simulink library "halin"  (R2021b)
settings: Solver=VariableStepAuto  StartTime=0.0  StopTime=10.0  RelTol=1e-3
undefined symbols (not defined in the file): TRUE
libraries: FVT_lib x177, hcu_lib x55
(part 11 of 17)

== system halin/HAL_IN/CAN4/ZONE_L1 ==
  DT_CAN4_SG_ZONE_L1 : Inport
  ZLDSEATAntiSta : Subsystem
  ZLDSEATEntryFunSta : Subsystem
  ZLDSEATErrorSta : Subsystem
  ZLDSEATMemSetSta : Subsystem
  ZLDSEATModeSta : Subsystem
  ZLDSEATVentSta : Subsystem
  ZLDSEATheaterSta : Subsystem
  bus_selector : BusSelector  OutputSignals=CAN4_ZL_DSEAT_Anti_Sta
  bus_selector1 : BusSelector  OutputSignals=CAN4_ZL_DSEAT_EntryFun_Sta
  bus_selector2 : BusSelector  OutputSignals=CAN4_ZL_DSEAT_Error_Sta
  bus_selector3 : BusSelector  OutputSignals=CAN4_ZL_DSEAT_MemSet_Sta
  bus_selector4 : BusSelector  OutputSignals=CAN4_ZL_DSEAT_Mode_Sta
  bus_selector5 : BusSelector  OutputSignals=CAN4_ZL_DSEAT_Vent_Sta
  bus_selector6 : BusSelector  OutputSignals=CAN4_ZL_DSEAT_heater_Sta
  VHAL_ZLDSEATAntiSta_flg : Outport
  VHAL_ZLDSEATEntryFunSta_flg : Outport  Port=2
  VHAL_ZLDSEATErrorSta_flg : Outport  Port=3
  VHAL_ZLDSEATMemSetSta_enum : Outport  Port=4
  VHAL_ZLDSEATModeSta_enum : Outport  Port=5
  VHAL_ZLDSEATVentSta_enum : Outport  Port=6
  VHAL_ZLDSEATheaterSta_enum : Outport  Port=7
  wires:
  DT_CAN4_SG_ZONE_L1/1 -> [DT_CAN4_SG_ZONE_L1]
  [DT_CAN4_SG_ZONE_L1] -> bus_selector/1
  bus_selector/1 -> ZLDSEATAntiSta/1(ZL_DSEAT_Anti_Sta)  "<CAN4_ZL_DSEAT_Anti_Sta>"
  ZLDSEATAntiSta/1(VHAL_ZLDSEATAntiSta_flg) -> VHAL_ZLDSEATAntiSta_flg/1
  [DT_CAN4_SG_ZONE_L1] -> bus_selector1/1
  bus_selector1/1 -> ZLDSEATEntryFunSta/1(ZL_DSEAT_EntryFun_Sta)  "<CAN4_ZL_DSEAT_EntryFun_Sta>"
  ZLDSEATEntryFunSta/1(VHAL_ZLDSEATEntryFunSta_flg) -> VHAL_ZLDSEATEntryFunSta_flg/1
  [DT_CAN4_SG_ZONE_L1] -> bus_selector2/1
  bus_selector2/1 -> ZLDSEATErrorSta/1(ZL_DSEAT_Error_Sta)  "<CAN4_ZL_DSEAT_Error_Sta>"
  ZLDSEATErrorSta/1(VHAL_ZLDSEATErrorSta_flg) -> VHAL_ZLDSEATErrorSta_flg/1
  [DT_CAN4_SG_ZONE_L1] -> bus_selector3/1
  bus_selector3/1 -> ZLDSEATMemSetSta/1(ZL_DSEAT_MemSet_Sta)  "<CAN4_ZL_DSEAT_MemSet_Sta>"
  ZLDSEATMemSetSta/1(VHAL_ZLDSEATMemSetSta_enum) -> VHAL_ZLDSEATMemSetSta_enum/1
  [DT_CAN4_SG_ZONE_L1] -> bus_selector4/1
  bus_selector4/1 -> ZLDSEATModeSta/1(ZL_DSEAT_Mode_Sta)  "<CAN4_ZL_DSEAT_Mode_Sta>"
  ZLDSEATModeSta/1(VHAL_ZLDSEATModeSta_enum) -> VHAL_ZLDSEATModeSta_enum/1
  [DT_CAN4_SG_ZONE_L1] -> bus_selector5/1
  bus_selector5/1 -> ZLDSEATVentSta/1(ZL_DSEAT_Vent_Sta)  "<CAN4_ZL_DSEAT_Vent_Sta>"
  ZLDSEATVentSta/1(VHAL_ZLDSEATVentSta_enum) -> VHAL_ZLDSEATVentSta_enum/1
  [DT_CAN4_SG_ZONE_L1] -> bus_selector6/1
  bus_selector6/1 -> ZLDSEATheaterSta/1(ZL_DSEAT_heater_Sta)  "<CAN4_ZL_DSEAT_heater_Sta>"
  ZLDSEATheaterSta/1(VHAL_ZLDSEATheaterSta_enum) -> VHAL_ZLDSEATheaterSta_enum/1

== system halin/HAL_IN/CAN4/ZONE_L2 ==
  DT_CAN4_SG_ZONE_L2 : Inport
  ZLAPMWinLFOpenedSta : Subsystem
  ZLAPMWinLROpenedSta : Subsystem
  bus_selector : BusSelector  OutputSignals=CAN4_ZL_APM_WinLFOpened_Sta
  bus_selector1 : BusSelector  OutputSignals=CAN4_ZL_APM_WinLROpened_Sta
  VHAL_ZLAPMWinLFOpenedSta_pct : Outport
  VHAL_ZLAPMWinLROpenedSta_pct : Outport  Port=2
  wires:
  DT_CAN4_SG_ZONE_L2/1 -> [DT_CAN4_SG_ZONE_L2]
  [DT_CAN4_SG_ZONE_L2] -> bus_selector/1
  bus_selector/1 -> ZLAPMWinLFOpenedSta/1(ZL_APM_WinLFOpened_Sta)  "<CAN4_ZL_APM_WinLFOpened_Sta>"
  ZLAPMWinLFOpenedSta/1(VHAL_ZLAPMWinLFOpenedSta_pct) -> VHAL_ZLAPMWinLFOpenedSta_pct/1
  [DT_CAN4_SG_ZONE_L2] -> bus_selector1/1
  bus_selector1/1 -> ZLAPMWinLROpenedSta/1(ZL_APM_WinLROpened_Sta)  "<CAN4_ZL_APM_WinLROpened_Sta>"
  ZLAPMWinLROpenedSta/1(VHAL_ZLAPMWinLROpenedSta_pct) -> VHAL_ZLAPMWinLROpenedSta_pct/1

== system halin/HAL_IN/CAN4/ZONE_R1 ==
  DT_CAN4_SG_ZONE_R1 : Inport
  ZRPSEATErrorSta : Subsystem
  ZRPSEATModeSta : Subsystem
  ZRPSEATVentSta : Subsystem
  ZRPSEATheaterSta : Subsystem
  ZRPTGActiveSta : Subsystem
  ZRPTGExistSta : Subsystem
  ZRPTGIsSetHeightSta : Subsystem
  ZRPTGSysSta : Subsystem
  bus_selector : BusSelector  OutputSignals=CAN4_ZR_PSEAT_Error_Sta
  bus_selector1 : BusSelector  OutputSignals=CAN4_ZR_PSEAT_Mode_Sta
  bus_selector2 : BusSelector  OutputSignals=CAN4_ZR_PSEAT_Vent_Sta
  bus_selector3 : BusSelector  OutputSignals=CAN4_ZR_PSEAT_heater_Sta
  bus_selector4 : BusSelector  OutputSignals=CAN4_ZR_PTG_Active_Sta
  bus_selector5 : BusSelector  OutputSignals=CAN4_ZR_PTG_Exist_Sta
  bus_selector6 : BusSelector  OutputSignals=CAN4_ZR_PTG_IsSetHeight_Sta
  bus_selector7 : BusSelector  OutputSignals=CAN4_ZR_PTG_Sys_Sta
  VHAL_ZRPSEATErrorSta_flg : Outport
  VHAL_ZRPSEATModeSta_enum : Outport  Port=2
  VHAL_ZRPSEATVentSta_enum : Outport  Port=3
  VHAL_ZRPSEATheaterSta_enum : Outport  Port=4
  VHAL_ZRPTGActiveSta_enum : Outport  Port=5
  VHAL_ZRPTGExistSta_flg : Outport  Port=6
  VHAL_ZRPTGIsSetHeightSta_flg : Outport  Port=7
  VHAL_ZRPTGSysSta_enum : Outport  Port=8
  wires:
  DT_CAN4_SG_ZONE_R1/1 -> [DT_CAN4_SG_ZONE_R1]
  [DT_CAN4_SG_ZONE_R1] -> bus_selector/1
  bus_selector/1 -> ZRPSEATErrorSta/1(ZR_PSEAT_Error_Sta)  "<CAN4_ZR_PSEAT_Error_Sta>"
  ZRPSEATErrorSta/1(VHAL_ZRPSEATErrorSta_flg) -> VHAL_ZRPSEATErrorSta_flg/1
  [DT_CAN4_SG_ZONE_R1] -> bus_selector1/1
  bus_selector1/1 -> ZRPSEATModeSta/1(ZR_PSEAT_Mode_Sta)  "<CAN4_ZR_PSEAT_Mode_Sta>"
  ZRPSEATModeSta/1(VHAL_ZRPSEATModeSta_enum) -> VHAL_ZRPSEATModeSta_enum/1
  [DT_CAN4_SG_ZONE_R1] -> bus_selector2/1
  bus_selector2/1 -> ZRPSEATVentSta/1(ZR_PSEAT_Vent_Sta)  "<CAN4_ZR_PSEAT_Vent_Sta>"
  ZRPSEATVentSta/1(VHAL_ZRPSEATVentSta_enum) -> VHAL_ZRPSEATVentSta_enum/1
  [DT_CAN4_SG_ZONE_R1] -> bus_selector3/1
  bus_selector3/1 -> ZRPSEATheaterSta/1(ZR_PSEAT_heater_Sta)  "<CAN4_ZR_PSEAT_heater_Sta>"
  ZRPSEATheaterSta/1(VHAL_ZRPSEATheaterSta_enum) -> VHAL_ZRPSEATheaterSta_enum/1
  [DT_CAN4_SG_ZONE_R1] -> bus_selector4/1
  bus_selector4/1 -> ZRPTGActiveSta/1(ZR_PTG_Active_Sta)  "<CAN4_ZR_PTG_Active_Sta>"
  ZRPTGActiveSta/1(VHAL_ZRPTGActiveSta_enum) -> VHAL_ZRPTGActiveSta_enum/1
  [DT_CAN4_SG_ZONE_R1] -> bus_selector5/1
  bus_selector5/1 -> ZRPTGExistSta/1(ZR_PTG_Exist_Sta)  "<CAN4_ZR_PTG_Exist_Sta>"
  ZRPTGExistSta/1(VHAL_ZRPTGExistSta_flg) -> VHAL_ZRPTGExistSta_flg/1
  [DT_CAN4_SG_ZONE_R1] -> bus_selector6/1
  bus_selector6/1 -> ZRPTGIsSetHeightSta/1(ZR_PTG_IsSetHeight_Sta)  "<CAN4_ZR_PTG_IsSetHeight_Sta>"
  ZRPTGIsSetHeightSta/1(VHAL_ZRPTGIsSetHeightSta_flg) -> VHAL_ZRPTGIsSetHeightSta_flg/1
  [DT_CAN4_SG_ZONE_R1] -> bus_selector7/1
  bus_selector7/1 -> ZRPTGSysSta/1(ZR_PTG_Sys_Sta)  "<CAN4_ZR_PTG_Sys_Sta>"
  ZRPTGSysSta/1(VHAL_ZRPTGSysSta_enum) -> VHAL_ZRPTGSysSta_enum/1

== system halin/HAL_IN/CAN4/ZONE_R2 ==
  DT_CAN4_SG_ZONE_R2 : Inport
  ZRAPMWinRFOpenedSta : Subsystem
  ZRAPMWinRROpenedSta : Subsystem
  ZRSEATLVentSta : Subsystem
  ZRSEATMLVentSta : Subsystem
  ZRSEATMRVentSta : Subsystem
  ZRSEATRVentSta : Subsystem
  bus_selector : BusSelector  OutputSignals=CAN4_ZR_APM_WinRFOpened_Sta
  bus_selector1 : BusSelector  OutputSignals=CAN4_ZR_APM_WinRROpened_Sta
  bus_selector2 : BusSelector  OutputSignals=CAN4_ZR_SEAT_LVent_Sta
  bus_selector3 : BusSelector  OutputSignals=CAN4_ZR_SEAT_MLVent_Sta
  bus_selector4 : BusSelector  OutputSignals=CAN4_ZR_SEAT_MRVent_Sta
  bus_selector5 : BusSelector  OutputSignals=CAN4_ZR_SEAT_RVent_Sta
  VHAL_ZRAPMWinRFOpenedSta_pct : Outport
  VHAL_ZRAPMWinRROpenedSta_pct : Outport  Port=2
  VHAL_ZRSEATLVentSta_enum : Outport  Port=3
  VHAL_ZRSEATMLVentSta_enum : Outport  Port=4
  VHAL_ZRSEATMRVentSta_enum : Outport  Port=5
  VHAL_ZRSEATRVentSta_enum : Outport  Port=6
  wires:
  DT_CAN4_SG_ZONE_R2/1 -> [DT_CAN4_SG_ZONE_R2]
  [DT_CAN4_SG_ZONE_R2] -> bus_selector/1
  bus_selector/1 -> ZRAPMWinRFOpenedSta/1(ZR_APM_WinRFOpened_Sta)  "<CAN4_ZR_APM_WinRFOpened_Sta>"
  ZRAPMWinRFOpenedSta/1(VHAL_ZRAPMWinRFOpenedSta_pct) -> VHAL_ZRAPMWinRFOpenedSta_pct/1
  [DT_CAN4_SG_ZONE_R2] -> bus_selector1/1
  bus_selector1/1 -> ZRAPMWinRROpenedSta/1(ZR_APM_WinRROpened_Sta)  "<CAN4_ZR_APM_WinRROpened_Sta>"
  ZRAPMWinRROpenedSta/1(VHAL_ZRAPMWinRROpenedSta_pct) -> VHAL_ZRAPMWinRROpenedSta_pct/1
  [DT_CAN4_SG_ZONE_R2] -> bus_selector2/1
  bus_selector2/1 -> ZRSEATLVentSta/1(ZR_SEAT_LVent_Sta)  "<CAN4_ZR_SEAT_LVent_Sta>"
  ZRSEATLVentSta/1(VHAL_ZRSEATLVentSta_enum) -> VHAL_ZRSEATLVentSta_enum/1
  [DT_CAN4_SG_ZONE_R2] -> bus_selector3/1
  bus_selector3/1 -> ZRSEATMLVentSta/1(ZR_SEAT_MLVent_Sta)  "<CAN4_ZR_SEAT_MLVent_Sta>"
  ZRSEATMLVentSta/1(VHAL_ZRSEATMLVentSta_enum) -> VHAL_ZRSEATMLVentSta_enum/1
  [DT_CAN4_SG_ZONE_R2] -> bus_selector4/1
  bus_selector4/1 -> ZRSEATMRVentSta/1(ZR_SEAT_MRVent_Sta)  "<CAN4_ZR_SEAT_MRVent_Sta>"
  ZRSEATMRVentSta/1(VHAL_ZRSEATMRVentSta_enum) -> VHAL_ZRSEATMRVentSta_enum/1
  [DT_CAN4_SG_ZONE_R2] -> bus_selector5/1
  bus_selector5/1 -> ZRSEATRVentSta/1(ZR_SEAT_RVent_Sta)  "<CAN4_ZR_SEAT_RVent_Sta>"
  ZRSEATRVentSta/1(VHAL_ZRSEATRVentSta_enum) -> VHAL_ZRSEATRVentSta_enum/1

== system halin/HAL_IN/CAN4/zGW_APTC1 ==
  DT_CAN4_SG_zGW_APTC1 : Inport
  FrntPTCLeActHeatPwr : Subsystem
  FrntPTCRearLeActHeatPwr : Subsystem
  FrntPTCRearRiActHeatPwr : Subsystem
  FrntPTCRiActHeatPwr : Subsystem
  bus_selector : BusSelector  OutputSignals=CAN4_FrntPTCLeActHeatPwr
  bus_selector1 : BusSelector  OutputSignals=CAN4_FrntPTCRearLeActHeatPwr
  bus_selector2 : BusSelector  OutputSignals=CAN4_FrntPTCRearRiActHeatPwr
  bus_selector3 : BusSelector  OutputSignals=CAN4_FrntPTCRiActHeatPwr
  VHAL_FrntPTCLeActHeatPwr_W : Outport
  VHAL_FrntPTCRearLeActHeatPwr_W : Outport  Port=2
  VHAL_FrntPTCRearRiActHeatPwr_W : Outport  Port=3
  VHAL_FrntPTCRiActHeatPwr_W : Outport  Port=4
  wires:
  DT_CAN4_SG_zGW_APTC1/1 -> [DT_CAN4_SG_zGW_APTC1]
  [DT_CAN4_SG_zGW_APTC1] -> bus_selector/1
  bus_selector/1 -> FrntPTCLeActHeatPwr/1(FrntPTCLeActHeatPwr)  "<CAN4_FrntPTCLeActHeatPwr>"
  FrntPTCLeActHeatPwr/1(VHAL_FrntPTCLeActHeatPwr_W) -> VHAL_FrntPTCLeActHeatPwr_W/1
  [DT_CAN4_SG_zGW_APTC1] -> bus_selector1/1
  bus_selector1/1 -> FrntPTCRearLeActHeatPwr/1(FrntPTCRearLeActHeatPwr)  "<CAN4_FrntPTCRearLeActHeatPwr>"
  FrntPTCRearLeActHeatPwr/1(VHAL_FrntPTCRearLeActHeatPwr_W) -> VHAL_FrntPTCRearLeActHeatPwr_W/1
  [DT_CAN4_SG_zGW_APTC1] -> bus_selector2/1
  bus_selector2/1 -> FrntPTCRearRiActHeatPwr/1(FrntPTCRearRiActHeatPwr)  "<CAN4_FrntPTCRearRiActHeatPwr>"
  FrntPTCRearRiActHeatPwr/1(VHAL_FrntPTCRearRiActHeatPwr_W) -> VHAL_FrntPTCRearRiActHeatPwr_W/1
  [DT_CAN4_SG_zGW_APTC1] -> bus_selector3/1
  bus_selector3/1 -> FrntPTCRiActHeatPwr/1(FrntPTCRiActHeatPwr)  "<CAN4_FrntPTCRiActHeatPwr>"
  FrntPTCRiActHeatPwr/1(VHAL_FrntPTCRiActHeatPwr_W) -> VHAL_FrntPTCRiActHeatPwr_W/1

== system halin/HAL_IN/CAN4/zGW_CANFr1 ==
  DT_CAN4_SG_zGW_CANFr1 : Inport
  COMPActualPwr : Subsystem
  COMPConCur : Subsystem
  COMPConVolt : Subsystem
  COMPStatorSpd : Subsystem
  PTC1PowerConsumption : Subsystem
  PTCActuPwrHSC6 : Subsystem
  bus_selector : BusSelector  OutputSignals=CAN4_COMP_ActualPwr
  bus_selector1 : BusSelector  OutputSignals=CAN4_COMP_ConCur
  bus_selector2 : BusSelector  OutputSignals=CAN4_COMP_ConVolt
  bus_selector3 : BusSelector  OutputSignals=CAN4_COMP_StatorSpd
  bus_selector4 : BusSelector  OutputSignals=CAN4_PTC1_PowerConsumption
  bus_selector5 : BusSelector  OutputSignals=CAN4_PTCActuPwrHSC6
  VHAL_COMPActualPwr_W : Outport
  VHAL_COMPConCur_A : Outport  Port=2
  VHAL_COMPConVolt_V : Outport  Port=3
  VHAL_COMPStatorSpd_rpm : Outport  Port=4
  VHAL_PTC1PowerConsumption_kW : Outport  Port=5
  VHAL_PTCActuPwrHSC6_enum : Outport  Port=6
  wires:
  DT_CAN4_SG_zGW_CANFr1/1 -> [DT_CAN4_SG_zGW_CANFr1]
  [DT_CAN4_SG_zGW_CANFr1] -> bus_selector/1
  bus_selector/1 -> COMPActualPwr/1(COMP_ActualPwr)  "<CAN4_COMP_ActualPwr>"
  COMPActualPwr/1(VHAL_COMPActualPwr_W) -> VHAL_COMPActualPwr_W/1
  [DT_CAN4_SG_zGW_CANFr1] -> bus_selector1/1
  bus_selector1/1 -> COMPConCur/1(COMP_ConCur)  "<CAN4_COMP_ConCur>"
  COMPConCur/1(VHAL_COMPConCur_A) -> VHAL_COMPConCur_A/1
  [DT_CAN4_SG_zGW_CANFr1] -> bus_selector2/1
  bus_selector2/1 -> COMPConVolt/1(COMP_ConVolt)  "<CAN4_COMP_ConVolt>"
  COMPConVolt/1(VHAL_COMPConVolt_V) -> VHAL_COMPConVolt_V/1
  [DT_CAN4_SG_zGW_CANFr1] -> bus_selector3/1
  bus_selector3/1 -> COMPStatorSpd/1(COMP_StatorSpd)  "<CAN4_COMP_StatorSpd>"
  COMPStatorSpd/1(VHAL_COMPStatorSpd_rpm) -> VHAL_COMPStatorSpd_rpm/1
  [DT_CAN4_SG_zGW_CANFr1] -> bus_selector4/1
  bus_selector4/1 -> PTC1PowerConsumption/1(PTC1_PowerConsumption)  "<CAN4_PTC1_PowerConsumption>"
  PTC1PowerConsumption/1(VHAL_PTC1PowerConsumption_kW) -> VHAL_PTC1PowerConsumption_kW/1
  [DT_CAN4_SG_zGW_CANFr1] -> bus_selector5/1
  bus_selector5/1 -> PTCActuPwrHSC6/1(PTCActuPwrHSC6)  "<CAN4_PTCActuPwrHSC6>"
  PTCActuPwrHSC6/1(VHAL_PTCActuPwrHSC6_enum) -> VHAL_PTCActuPwrHSC6_enum/1

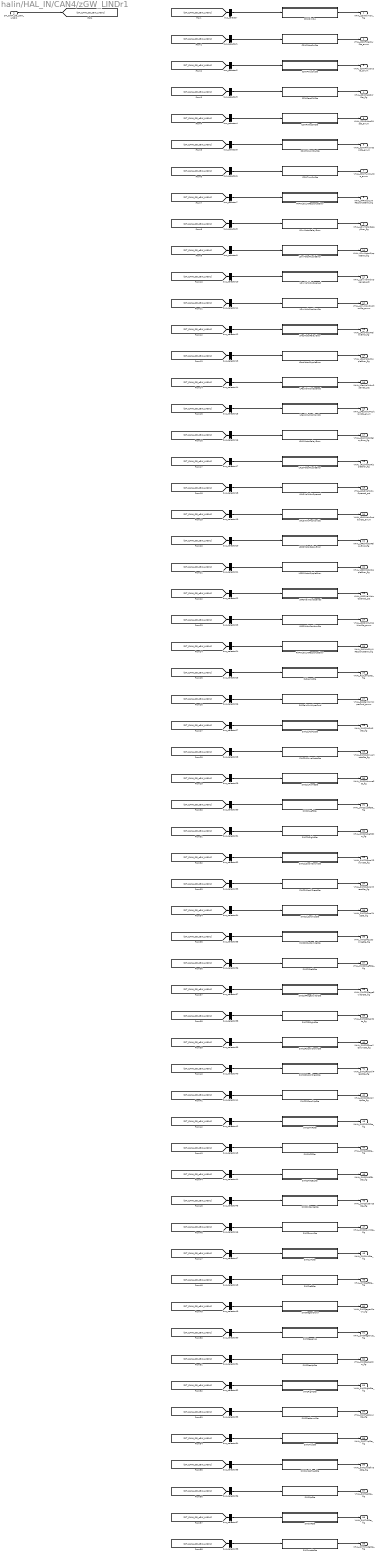
== system halin/HAL_IN/CAN4/zGW_LINDr1 ==
  DT_CAN4_SG_zGW_LINDr1 : Inport
  CSWDimSw : Subsystem
  CSWFWasSwSta : Subsystem
  CSWFWipSwSta : Subsystem
  CSWPassSWSta : Subsystem
  CSWRWasSWSta : Subsystem
  CSWRWipIntSwSta : Subsystem
  CSWTurnSwSta : Subsystem
  FAPWL01LINResponseError : Subsystem
  LDrvMotorRelayError : Subsystem
  LDrvMotorRippleError : Subsystem
  LDrvValWdwOpened : Subsystem
  LDrvWdwPositionSts : Subsystem
  LPasMotorRelayError : Subsystem
  LPasMotorRippleError : Subsystem
  LPasValWdwOpened : Subsystem
  LPasWdwPositionSts : Subsystem
  LRLDMotorRelayError : Subsystem
  LRLDMotorRippleError : Subsystem
  LRLDValWdwOpened : Subsystem
  LRLDWdwPositionSts : Subsystem
  LRRDMotorRelayError : Subsystem
  LRRDMotorRippleError : Subsystem
  LRRDValWdwOpened : Subsystem
  LRRDWdwPositionSts : Subsystem
  RAPWL01LINResponseError : Subsystem
  RLSLampSta : Subsystem
  RLSRainSnrWiperCmd : Subsystem
  SWC2LADASSta : Subsystem
  SWC2LDriveModeSta : Subsystem
  SWC2LHomeSta : Subsystem
  SWC2LLeftSta : Subsystem
  SWC2LRightSta : Subsystem
  SWC2LScrollDownSta : Subsystem
  SWC2LScrollPressSta : Subsystem
  SWC2LScrollUpSta : Subsystem
  SWC2RCustomizeSta : Subsystem
  SWC2RLeftSta : Subsystem
  SWC2RPageSwitchSta : Subsystem
  SWC2RRightSta : Subsystem
  SWC2RScrollDownSta : Subsystem
  SWC2RScrollPressSta : Subsystem
  SWC2RScrollUpSta : Subsystem
  SWC2RVRSta : Subsystem
  SWCACCSta : Subsystem
  SWCCANCELSta : Subsystem
  SWCDistanceSta : Subsystem
  SWCDownSta : Subsystem
  SWCLKASta : Subsystem
  SWCLeftSta : Subsystem
  SWCRegenDown : Subsystem
  SWCRegenUp : Subsystem
  SWCResUpSta : Subsystem
  SWCRightSta : Subsystem
  SWCSetdownSta : Subsystem
  SWCTripSta : Subsystem
  SWCUndefinedSta : Subsystem
  SWCUpSta : Subsystem
  SWCVRSta : Subsystem
  SWCmodeSta : Subsystem
  bus_selector : BusSelector  OutputSignals=CAN4_CSW_DimSw
  bus_selector1 : BusSelector  OutputSignals=CAN4_CSW_FWasSw_Sta
  bus_selector10 : BusSelector  OutputSignals=CAN4_L_Drv_Val_Wdw_Opened
  bus_selector11 : BusSelector  OutputSignals=CAN4_L_Drv_Wdw_PositionSts
  bus_selector12 : BusSelector  OutputSignals=CAN4_L_Pas_Motor_Relay_Error
  bus_selector13 : BusSelector  OutputSignals=CAN4_L_Pas_Motor_Ripple_Error
  bus_selector14 : BusSelector  OutputSignals=CAN4_L_Pas_Val_Wdw_Opened
  bus_selector15 : BusSelector  OutputSignals=CAN4_L_Pas_Wdw_PositionSts
  bus_selector16 : BusSelector  OutputSignals=CAN4_L_RLD_Motor_Relay_Error
  bus_selector17 : BusSelector  OutputSignals=CAN4_L_RLD_Motor_Ripple_Error
  bus_selector18 : BusSelector  OutputSignals=CAN4_L_RLD_Val_Wdw_Opened
  bus_selector19 : BusSelector  OutputSignals=CAN4_L_RLD_Wdw_PositionSts
  bus_selector2 : BusSelector  OutputSignals=CAN4_CSW_FWipSw_Sta
  bus_selector20 : BusSelector  OutputSignals=CAN4_L_RRD_Motor_Relay_Error
  bus_selector21 : BusSelector  OutputSignals=CAN4_L_RRD_Motor_Ripple_Error
  bus_selector22 : BusSelector  OutputSignals=CAN4_L_RRD_Val_Wdw_Opened
  bus_selector23 : BusSelector  OutputSignals=CAN4_L_RRD_Wdw_PositionSts
  bus_selector24 : BusSelector  OutputSignals=CAN4_RAPWL_01_LIN_Response_Error
  bus_selector25 : BusSelector  OutputSignals=CAN4_RLS_Lamp_Sta
  bus_selector26 : BusSelector  OutputSignals=CAN4_RLS_RainSnrWiperCmd
  bus_selector27 : BusSelector  OutputSignals=CAN4_SWC2_L_ADAS_Sta
  bus_selector28 : BusSelector  OutputSignals=CAN4_SWC2_L_DriveMode_Sta
  bus_selector29 : BusSelector  OutputSignals=CAN4_SWC2_L_Home_Sta
  bus_selector3 : BusSelector  OutputSignals=CAN4_CSW_PassSW_Sta
  bus_selector30 : BusSelector  OutputSignals=CAN4_SWC2_L_Left_Sta
  bus_selector31 : BusSelector  OutputSignals=CAN4_SWC2_L_Right_Sta
  bus_selector32 : BusSelector  OutputSignals=CAN4_SWC2_L_ScrollDown_Sta
  bus_selector33 : BusSelector  OutputSignals=CAN4_SWC2_L_ScrollPress_Sta
  bus_selector34 : BusSelector  OutputSignals=CAN4_SWC2_L_ScrollUp_Sta
  bus_selector35 : BusSelector  OutputSignals=CAN4_SWC2_R_Customize_Sta
  bus_selector36 : BusSelector  OutputSignals=CAN4_SWC2_R_Left_Sta
  bus_selector37 : BusSelector  OutputSignals=CAN4_SWC2_R_PageSwitch_Sta
  bus_selector38 : BusSelector  OutputSignals=CAN4_SWC2_R_Right_Sta
  bus_selector39 : BusSelector  OutputSignals=CAN4_SWC2_R_ScrollDown_Sta
  bus_selector4 : BusSelector  OutputSignals=CAN4_CSW_RWasSW_Sta
  bus_selector40 : BusSelector  OutputSignals=CAN4_SWC2_R_ScrollPress_Sta
  bus_selector41 : BusSelector  OutputSignals=CAN4_SWC2_R_ScrollUp_Sta
  bus_selector42 : BusSelector  OutputSignals=CAN4_SWC2_R_VR_Sta
  bus_selector43 : BusSelector  OutputSignals=CAN4_SWC_ACC_Sta
  bus_selector44 : BusSelector  OutputSignals=CAN4_SWC_CANCEL_Sta
  bus_selector45 : BusSelector  OutputSignals=CAN4_SWC_Distance_Sta
  bus_selector46 : BusSelector  OutputSignals=CAN4_SWC_Down_Sta
  bus_selector47 : BusSelector  OutputSignals=CAN4_SWC_LKA_Sta
  bus_selector48 : BusSelector  OutputSignals=CAN4_SWC_Left_Sta
  bus_selector49 : BusSelector  OutputSignals=CAN4_SWC_RegenDown
  bus_selector5 : BusSelector  OutputSignals=CAN4_CSW_RWipIntSw_Sta
  bus_selector50 : BusSelector  OutputSignals=CAN4_SWC_RegenUp
  bus_selector51 : BusSelector  OutputSignals=CAN4_SWC_Res_Up_Sta
  bus_selector52 : BusSelector  OutputSignals=CAN4_SWC_Right_Sta
  bus_selector53 : BusSelector  OutputSignals=CAN4_SWC_Set_down_Sta
  bus_selector54 : BusSelector  OutputSignals=CAN4_SWC_Trip_Sta
  bus_selector55 : BusSelector  OutputSignals=CAN4_SWC_Undefined_Sta
  bus_selector56 : BusSelector  OutputSignals=CAN4_SWC_Up_Sta
  bus_selector57 : BusSelector  OutputSignals=CAN4_SWC_VR_Sta
  bus_selector58 : BusSelector  OutputSignals=CAN4_SWC_mode_Sta
  bus_selector6 : BusSelector  OutputSignals=CAN4_CSW_TurnSw_Sta
  bus_selector7 : BusSelector  OutputSignals=CAN4_FAPWL_01_LIN_Response_Error
  bus_selector8 : BusSelector  OutputSignals=CAN4_L_Drv_Motor_Relay_Error
  bus_selector9 : BusSelector  OutputSignals=CAN4_L_Drv_Motor_Ripple_Error
  VHAL_CSWDimSw_flg : Outport
  VHAL_CSWFWasSwSta_enum : Outport  Port=2
  VHAL_CSWFWipSwSta_enum : Outport  Port=3
  VHAL_CSWPassSWSta_flg : Outport  Port=4
  VHAL_CSWRWasSWSta_enum : Outport  Port=5
  VHAL_CSWRWipIntSwSta_enum : Outport  Port=6
  VHAL_CSWTurnSwSta_enum : Outport  Port=7
  VHAL_FAPWL01LINResponseError_flg : Outport  Port=8
  VHAL_LDrvMotorRelayError_flg : Outport  Port=9
  VHAL_LDrvMotorRippleError_flg : Outport  Port=10
  VHAL_LDrvValWdwOpened_pct : Outport  Port=11
  VHAL_LDrvWdwPositionSts_enum : Outport  Port=12
  VHAL_LPasMotorRelayError_flg : Outport  Port=13
  VHAL_LPasMotorRippleError_flg : Outport  Port=14
  VHAL_LPasValWdwOpened_pct : Outport  Port=15
  VHAL_LPasWdwPositionSts_enum : Outport  Port=16
  VHAL_LRLDMotorRelayError_flg : Outport  Port=17
  VHAL_LRLDMotorRippleError_flg : Outport  Port=18
  VHAL_LRLDValWdwOpened_pct : Outport  Port=19
  VHAL_LRLDWdwPositionSts_enum : Outport  Port=20
  VHAL_LRRDMotorRelayError_flg : Outport  Port=21
  VHAL_LRRDMotorRippleError_flg : Outport  Port=22
  VHAL_LRRDValWdwOpened_pct : Outport  Port=23
  VHAL_LRRDWdwPositionSts_enum : Outport  Port=24
  VHAL_RAPWL01LINResponseError_flg : Outport  Port=25
  VHAL_RLSLampSta_flg : Outport  Port=26
  VHAL_RLSRainSnrWiperCmd_enum : Outport  Port=27
  VHAL_SWC2LADASSta_flg : Outport  Port=28
  VHAL_SWC2LDriveModeSta_flg : Outport  Port=29
  VHAL_SWC2LHomeSta_flg : Outport  Port=30
  VHAL_SWC2LLeftSta_flg : Outport  Port=31
  VHAL_SWC2LRightSta_flg : Outport  Port=32
  VHAL_SWC2LScrollDownSta_flg : Outport  Port=33
  VHAL_SWC2LScrollPressSta_flg : Outport  Port=34
  VHAL_SWC2LScrollUpSta_flg : Outport  Port=35
  VHAL_SWC2RCustomizeSta_flg : Outport  Port=36
  VHAL_SWC2RLeftSta_flg : Outport  Port=37
  VHAL_SWC2RPageSwitchSta_flg : Outport  Port=38
  VHAL_SWC2RRightSta_flg : Outport  Port=39
  VHAL_SWC2RScrollDownSta_flg : Outport  Port=40
  VHAL_SWC2RScrollPressSta_flg : Outport  Port=41
  VHAL_SWC2RScrollUpSta_flg : Outport  Port=42
  VHAL_SWC2RVRSta_flg : Outport  Port=43
  VHAL_SWCACCSta_flg : Outport  Port=44
  VHAL_SWCCANCELSta_flg : Outport  Port=45
  VHAL_SWCDistanceSta_flg : Outport  Port=46
  VHAL_SWCDownSta_flg : Outport  Port=47
  VHAL_SWCLKASta_flg : Outport  Port=48
  VHAL_SWCLeftSta_flg : Outport  Port=49
  VHAL_SWCRegenDown_flg : Outport  Port=50
  VHAL_SWCRegenUp_flg : Outport  Port=51
  VHAL_SWCResUpSta_flg : Outport  Port=52
  VHAL_SWCRightSta_flg : Outport  Port=53
  VHAL_SWCSetdownSta_flg : Outport  Port=54
  VHAL_SWCTripSta_flg : Outport  Port=55
  VHAL_SWCUndefinedSta_flg : Outport  Port=56
  VHAL_SWCUpSta_flg : Outport  Port=57
  VHAL_SWCVRSta_flg : Outport  Port=58
  VHAL_SWCmodeSta_flg : Outport  Port=59
  wires:
  DT_CAN4_SG_zGW_LINDr1/1 -> [DT_CAN4_SG_zGW_LINDr1]
  [DT_CAN4_SG_zGW_LINDr1] -> bus_selector/1
  bus_selector/1 -> CSWDimSw/1(CSW_DimSw)  "<CAN4_CSW_DimSw>"
  CSWDimSw/1(VHAL_CSWDimSw_flg) -> VHAL_CSWDimSw_flg/1
  [DT_CAN4_SG_zGW_LINDr1] -> bus_selector1/1
  bus_selector1/1 -> CSWFWasSwSta/1(CSW_FWasSw_Sta)  "<CAN4_CSW_FWasSw_Sta>"
  CSWFWasSwSta/1(VHAL_CSWFWasSwSta_enum) -> VHAL_CSWFWasSwSta_enum/1
  [DT_CAN4_SG_zGW_LINDr1] -> bus_selector2/1
  bus_selector2/1 -> CSWFWipSwSta/1(CSW_FWipSw_Sta)  "<CAN4_CSW_FWipSw_Sta>"
  CSWFWipSwSta/1(VHAL_CSWFWipSwSta_enum) -> VHAL_CSWFWipSwSta_enum/1
  [DT_CAN4_SG_zGW_LINDr1] -> bus_selector3/1
  bus_selector3/1 -> CSWPassSWSta/1(CSW_PassSW_Sta)  "<CAN4_CSW_PassSW_Sta>"
  CSWPassSWSta/1(VHAL_CSWPassSWSta_flg) -> VHAL_CSWPassSWSta_flg/1
  [DT_CAN4_SG_zGW_LINDr1] -> bus_selector4/1
  bus_selector4/1 -> CSWRWasSWSta/1(CSW_RWasSW_Sta)  "<CAN4_CSW_RWasSW_Sta>"
  CSWRWasSWSta/1(VHAL_CSWRWasSWSta_enum) -> VHAL_CSWRWasSWSta_enum/1
  [DT_CAN4_SG_zGW_LINDr1] -> bus_selector5/1
  bus_selector5/1 -> CSWRWipIntSwSta/1(CSW_RWipIntSw_Sta)  "<CAN4_CSW_RWipIntSw_Sta>"
  CSWRWipIntSwSta/1(VHAL_CSWRWipIntSwSta_enum) -> VHAL_CSWRWipIntSwSta_enum/1
  [DT_CAN4_SG_zGW_LINDr1] -> bus_selector6/1
  bus_selector6/1 -> CSWTurnSwSta/1(CSW_TurnSw_Sta)  "<CAN4_CSW_TurnSw_Sta>"
  CSWTurnSwSta/1(VHAL_CSWTurnSwSta_enum) -> VHAL_CSWTurnSwSta_enum/1
  [DT_CAN4_SG_zGW_LINDr1] -> bus_selector7/1
  bus_selector7/1 -> FAPWL01LINResponseError/1(FAPWL_01_LIN_Response_Error)  "<CAN4_FAPWL_01_LIN_Response_Error>"
  FAPWL01LINResponseError/1(VHAL_FAPWL01LINResponseError_flg) -> VHAL_FAPWL01LINResponseError_flg/1
  [DT_CAN4_SG_zGW_LINDr1] -> bus_selector8/1
  bus_selector8/1 -> LDrvMotorRelayError/1(L_Drv_Motor_Relay_Error)  "<CAN4_L_Drv_Motor_Relay_Error>"
  LDrvMotorRelayError/1(VHAL_LDrvMotorRelayError_flg) -> VHAL_LDrvMotorRelayError_flg/1
  [DT_CAN4_SG_zGW_LINDr1] -> bus_selector9/1
  bus_selector9/1 -> LDrvMotorRippleError/1(L_Drv_Motor_Ripple_Error)  "<CAN4_L_Drv_Motor_Ripple_Error>"
  LDrvMotorRippleError/1(VHAL_LDrvMotorRippleError_flg) -> VHAL_LDrvMotorRippleError_flg/1
  [DT_CAN4_SG_zGW_LINDr1] -> bus_selector10/1
  bus_selector10/1 -> LDrvValWdwOpened/1(L_Drv_Val_Wdw_Opened)  "<CAN4_L_Drv_Val_Wdw_Opened>"
  LDrvValWdwOpened/1(VHAL_LDrvValWdwOpened_pct) -> VHAL_LDrvValWdwOpened_pct/1
  [DT_CAN4_SG_zGW_LINDr1] -> bus_selector11/1
  bus_selector11/1 -> LDrvWdwPositionSts/1(L_Drv_Wdw_PositionSts)  "<CAN4_L_Drv_Wdw_PositionSts>"
  LDrvWdwPositionSts/1(VHAL_LDrvWdwPositionSts_enum) -> VHAL_LDrvWdwPositionSts_enum/1
  [DT_CAN4_SG_zGW_LINDr1] -> bus_selector12/1
  bus_selector12/1 -> LPasMotorRelayError/1(L_Pas_Motor_Relay_Error)  "<CAN4_L_Pas_Motor_Relay_Error>"
  LPasMotorRelayError/1(VHAL_LPasMotorRelayError_flg) -> VHAL_LPasMotorRelayError_flg/1
  [DT_CAN4_SG_zGW_LINDr1] -> bus_selector13/1
  bus_selector13/1 -> LPasMotorRippleError/1(L_Pas_Motor_Ripple_Error)  "<CAN4_L_Pas_Motor_Ripple_Error>"
  LPasMotorRippleError/1(VHAL_LPasMotorRippleError_flg) -> VHAL_LPasMotorRippleError_flg/1
  [DT_CAN4_SG_zGW_LINDr1] -> bus_selector14/1
  bus_selector14/1 -> LPasValWdwOpened/1(L_Pas_Val_Wdw_Opened)  "<CAN4_L_Pas_Val_Wdw_Opened>"
  LPasValWdwOpened/1(VHAL_LPasValWdwOpened_pct) -> VHAL_LPasValWdwOpened_pct/1
  [DT_CAN4_SG_zGW_LINDr1] -> bus_selector15/1
  bus_selector15/1 -> LPasWdwPositionSts/1(L_Pas_Wdw_PositionSts)  "<CAN4_L_Pas_Wdw_PositionSts>"
  LPasWdwPositionSts/1(VHAL_LPasWdwPositionSts_enum) -> VHAL_LPasWdwPositionSts_enum/1
  [DT_CAN4_SG_zGW_LINDr1] -> bus_selector16/1
  bus_selector16/1 -> LRLDMotorRelayError/1(L_RLD_Motor_Relay_Error)  "<CAN4_L_RLD_Motor_Relay_Error>"
  LRLDMotorRelayError/1(VHAL_LRLDMotorRelayError_flg) -> VHAL_LRLDMotorRelayError_flg/1
  [DT_CAN4_SG_zGW_LINDr1] -> bus_selector17/1
  bus_selector17/1 -> LRLDMotorRippleError/1(L_RLD_Motor_Ripple_Error)  "<CAN4_L_RLD_Motor_Ripple_Error>"
  LRLDMotorRippleError/1(VHAL_LRLDMotorRippleError_flg) -> VHAL_LRLDMotorRippleError_flg/1
  [DT_CAN4_SG_zGW_LINDr1] -> bus_selector18/1
  bus_selector18/1 -> LRLDValWdwOpened/1(L_RLD_Val_Wdw_Opened)  "<CAN4_L_RLD_Val_Wdw_Opened>"
  LRLDValWdwOpened/1(VHAL_LRLDValWdwOpened_pct) -> VHAL_LRLDValWdwOpened_pct/1
  [DT_CAN4_SG_zGW_LINDr1] -> bus_selector19/1
  bus_selector19/1 -> LRLDWdwPositionSts/1(L_RLD_Wdw_PositionSts)  "<CAN4_L_RLD_Wdw_PositionSts>"
  LRLDWdwPositionSts/1(VHAL_LRLDWdwPositionSts_enum) -> VHAL_LRLDWdwPositionSts_enum/1
  [DT_CAN4_SG_zGW_LINDr1] -> bus_selector20/1
  bus_selector20/1 -> LRRDMotorRelayError/1(L_RRD_Motor_Relay_Error)  "<CAN4_L_RRD_Motor_Relay_Error>"
  LRRDMotorRelayError/1(VHAL_LRRDMotorRelayError_flg) -> VHAL_LRRDMotorRelayError_flg/1
  [DT_CAN4_SG_zGW_LINDr1] -> bus_selector21/1
  bus_selector21/1 -> LRRDMotorRippleError/1(L_RRD_Motor_Ripple_Error)  "<CAN4_L_RRD_Motor_Ripple_Error>"
  LRRDMotorRippleError/1(VHAL_LRRDMotorRippleError_flg) -> VHAL_LRRDMotorRippleError_flg/1
  [DT_CAN4_SG_zGW_LINDr1] -> bus_selector22/1
  bus_selector22/1 -> LRRDValWdwOpened/1(L_RRD_Val_Wdw_Opened)  "<CAN4_L_RRD_Val_Wdw_Opened>"
  LRRDValWdwOpened/1(VHAL_LRRDValWdwOpened_pct) -> VHAL_LRRDValWdwOpened_pct/1
  [DT_CAN4_SG_zGW_LINDr1] -> bus_selector23/1
  bus_selector23/1 -> LRRDWdwPositionSts/1(L_RRD_Wdw_PositionSts)  "<CAN4_L_RRD_Wdw_PositionSts>"
  LRRDWdwPositionSts/1(VHAL_LRRDWdwPositionSts_enum) -> VHAL_LRRDWdwPositionSts_enum/1
  [DT_CAN4_SG_zGW_LINDr1] -> bus_selector24/1
  bus_selector24/1 -> RAPWL01LINResponseError/1(RAPWL_01_LIN_Response_Error)  "<CAN4_RAPWL_01_LIN_Response_Error>"
  RAPWL01LINResponseError/1(VHAL_RAPWL01LINResponseError_flg) -> VHAL_RAPWL01LINResponseError_flg/1
  [DT_CAN4_SG_zGW_LINDr1] -> bus_selector25/1
  bus_selector25/1 -> RLSLampSta/1(RLS_Lamp_Sta)  "<CAN4_RLS_Lamp_Sta>"
  RLSLampSta/1(VHAL_RLSLampSta_flg) -> VHAL_RLSLampSta_flg/1
  [DT_CAN4_SG_zGW_LINDr1] -> bus_selector26/1
  bus_selector26/1 -> RLSRainSnrWiperCmd/1(RLS_RainSnrWiperCmd)  "<CAN4_RLS_RainSnrWiperCmd>"
  RLSRainSnrWiperCmd/1(VHAL_RLSRainSnrWiperCmd_enum) -> VHAL_RLSRainSnrWiperCmd_enum/1
  [DT_CAN4_SG_zGW_LINDr1] -> bus_selector27/1
  bus_selector27/1 -> SWC2LADASSta/1(SWC2_L_ADAS_Sta)  "<CAN4_SWC2_L_ADAS_Sta>"
  SWC2LADASSta/1(VHAL_SWC2LADASSta_flg) -> VHAL_SWC2LADASSta_flg/1
  [DT_CAN4_SG_zGW_LINDr1] -> bus_selector28/1
  bus_selector28/1 -> SWC2LDriveModeSta/1(SWC2_L_DriveMode_Sta)  "<CAN4_SWC2_L_DriveMode_Sta>"
  SWC2LDriveModeSta/1(VHAL_SWC2LDriveModeSta_flg) -> VHAL_SWC2LDriveModeSta_flg/1
  [DT_CAN4_SG_zGW_LINDr1] -> bus_selector29/1
  bus_selector29/1 -> SWC2LHomeSta/1(SWC2_L_Home_Sta)  "<CAN4_SWC2_L_Home_Sta>"
  SWC2LHomeSta/1(VHAL_SWC2LHomeSta_flg) -> VHAL_SWC2LHomeSta_flg/1
  [DT_CAN4_SG_zGW_LINDr1] -> bus_selector30/1
  bus_selector30/1 -> SWC2LLeftSta/1(SWC2_L_Left_Sta)  "<CAN4_SWC2_L_Left_Sta>"
  SWC2LLeftSta/1(VHAL_SWC2LLeftSta_flg) -> VHAL_SWC2LLeftSta_flg/1
  [DT_CAN4_SG_zGW_LINDr1] -> bus_selector31/1
  bus_selector31/1 -> SWC2LRightSta/1(SWC2_L_Right_Sta)  "<CAN4_SWC2_L_Right_Sta>"
  SWC2LRightSta/1(VHAL_SWC2LRightSta_flg) -> VHAL_SWC2LRightSta_flg/1
  [DT_CAN4_SG_zGW_LINDr1] -> bus_selector32/1
  bus_selector32/1 -> SWC2LScrollDownSta/1(SWC2_L_ScrollDown_Sta)  "<CAN4_SWC2_L_ScrollDown_Sta>"
  SWC2LScrollDownSta/1(VHAL_SWC2LScrollDownSta_flg) -> VHAL_SWC2LScrollDownSta_flg/1
  [DT_CAN4_SG_zGW_LINDr1] -> bus_selector33/1
  bus_selector33/1 -> SWC2LScrollPressSta/1(SWC2_L_ScrollPress_Sta)  "<CAN4_SWC2_L_ScrollPress_Sta>"
  SWC2LScrollPressSta/1(VHAL_SWC2LScrollPressSta_flg) -> VHAL_SWC2LScrollPressSta_flg/1
  [DT_CAN4_SG_zGW_LINDr1] -> bus_selector34/1
  bus_selector34/1 -> SWC2LScrollUpSta/1(SWC2_L_ScrollUp_Sta)  "<CAN4_SWC2_L_ScrollUp_Sta>"
  SWC2LScrollUpSta/1(VHAL_SWC2LScrollUpSta_flg) -> VHAL_SWC2LScrollUpSta_flg/1
  [DT_CAN4_SG_zGW_LINDr1] -> bus_selector35/1
  bus_selector35/1 -> SWC2RCustomizeSta/1(SWC2_R_Customize_Sta)  "<CAN4_SWC2_R_Customize_Sta>"
  SWC2RCustomizeSta/1(VHAL_SWC2RCustomizeSta_flg) -> VHAL_SWC2RCustomizeSta_flg/1
  [DT_CAN4_SG_zGW_LINDr1] -> bus_selector36/1
  bus_selector36/1 -> SWC2RLeftSta/1(SWC2_R_Left_Sta)  "<CAN4_SWC2_R_Left_Sta>"
  SWC2RLeftSta/1(VHAL_SWC2RLeftSta_flg) -> VHAL_SWC2RLeftSta_flg/1
  [DT_CAN4_SG_zGW_LINDr1] -> bus_selector37/1
  bus_selector37/1 -> SWC2RPageSwitchSta/1(SWC2_R_PageSwitch_Sta)  "<CAN4_SWC2_R_PageSwitch_Sta>"
  SWC2RPageSwitchSta/1(VHAL_SWC2RPageSwitchSta_flg) -> VHAL_SWC2RPageSwitchSta_flg/1
  [DT_CAN4_SG_zGW_LINDr1] -> bus_selector38/1
  bus_selector38/1 -> SWC2RRightSta/1(SWC2_R_Right_Sta)  "<CAN4_SWC2_R_Right_Sta>"
  SWC2RRightSta/1(VHAL_SWC2RRightSta_flg) -> VHAL_SWC2RRightSta_flg/1
  [DT_CAN4_SG_zGW_LINDr1] -> bus_selector39/1
  bus_selector39/1 -> SWC2RScrollDownSta/1(SWC2_R_ScrollDown_Sta)  "<CAN4_SWC2_R_ScrollDown_Sta>"
  SWC2RScrollDownSta/1(VHAL_SWC2RScrollDownSta_flg) -> VHAL_SWC2RScrollDownSta_flg/1
  [DT_CAN4_SG_zGW_LINDr1] -> bus_selector40/1
  bus_selector40/1 -> SWC2RScrollPressSta/1(SWC2_R_ScrollPress_Sta)  "<CAN4_SWC2_R_ScrollPress_Sta>"
  SWC2RScrollPressSta/1(VHAL_SWC2RScrollPressSta_flg) -> VHAL_SWC2RScrollPressSta_flg/1
  [DT_CAN4_SG_zGW_LINDr1] -> bus_selector41/1
  bus_selector41/1 -> SWC2RScrollUpSta/1(SWC2_R_ScrollUp_Sta)  "<CAN4_SWC2_R_ScrollUp_Sta>"
  SWC2RScrollUpSta/1(VHAL_SWC2RScrollUpSta_flg) -> VHAL_SWC2RScrollUpSta_flg/1
  [DT_CAN4_SG_zGW_LINDr1] -> bus_selector42/1
  bus_selector42/1 -> SWC2RVRSta/1(SWC2_R_VR_Sta)  "<CAN4_SWC2_R_VR_Sta>"
  SWC2RVRSta/1(VHAL_SWC2RVRSta_flg) -> VHAL_SWC2RVRSta_flg/1
  [DT_CAN4_SG_zGW_LINDr1] -> bus_selector43/1
  bus_selector43/1 -> SWCACCSta/1(SWC_ACC_Sta)  "<CAN4_SWC_ACC_Sta>"
  SWCACCSta/1(VHAL_SWCACCSta_flg) -> VHAL_SWCACCSta_flg/1
  [DT_CAN4_SG_zGW_LINDr1] -> bus_selector44/1
  bus_selector44/1 -> SWCCANCELSta/1(SWC_CANCEL_Sta)  "<CAN4_SWC_CANCEL_Sta>"
  SWCCANCELSta/1(VHAL_SWCCANCELSta_flg) -> VHAL_SWCCANCELSta_flg/1
  [DT_CAN4_SG_zGW_LINDr1] -> bus_selector45/1
  bus_selector45/1 -> SWCDistanceSta/1(SWC_Distance_Sta)  "<CAN4_SWC_Distance_Sta>"
  SWCDistanceSta/1(VHAL_SWCDistanceSta_flg) -> VHAL_SWCDistanceSta_flg/1
  [DT_CAN4_SG_zGW_LINDr1] -> bus_selector46/1
  bus_selector46/1 -> SWCDownSta/1(SWC_Down_Sta)  "<CAN4_SWC_Down_Sta>"
  SWCDownSta/1(VHAL_SWCDownSta_flg) -> VHAL_SWCDownSta_flg/1
  [DT_CAN4_SG_zGW_LINDr1] -> bus_selector47/1
  bus_selector47/1 -> SWCLKASta/1(SWC_LKA_Sta)  "<CAN4_SWC_LKA_Sta>"
  SWCLKASta/1(VHAL_SWCLKASta_flg) -> VHAL_SWCLKASta_flg/1
  [DT_CAN4_SG_zGW_LINDr1] -> bus_selector48/1
  bus_selector48/1 -> SWCLeftSta/1(SWC_Left_Sta)  "<CAN4_SWC_Left_Sta>"
  SWCLeftSta/1(VHAL_SWCLeftSta_flg) -> VHAL_SWCLeftSta_flg/1
  [DT_CAN4_SG_zGW_LINDr1] -> bus_selector49/1
  bus_selector49/1 -> SWCRegenDown/1(SWC_RegenDown)  "<CAN4_SWC_RegenDown>"
  SWCRegenDown/1(VHAL_SWCRegenDown_flg) -> VHAL_SWCRegenDown_flg/1
  [DT_CAN4_SG_zGW_LINDr1] -> bus_selector50/1
  bus_selector50/1 -> SWCRegenUp/1(SWC_RegenUp)  "<CAN4_SWC_RegenUp>"
  SWCRegenUp/1(VHAL_SWCRegenUp_flg) -> VHAL_SWCRegenUp_flg/1
  [DT_CAN4_SG_zGW_LINDr1] -> bus_selector51/1
  bus_selector51/1 -> SWCResUpSta/1(SWC_Res_Up_Sta)  "<CAN4_SWC_Res_Up_Sta>"
  SWCResUpSta/1(VHAL_SWCResUpSta_flg) -> VHAL_SWCResUpSta_flg/1
  [DT_CAN4_SG_zGW_LINDr1] -> bus_selector52/1
  bus_selector52/1 -> SWCRightSta/1(SWC_Right_Sta)  "<CAN4_SWC_Right_Sta>"
  SWCRightSta/1(VHAL_SWCRightSta_flg) -> VHAL_SWCRightSta_flg/1
  [DT_CAN4_SG_zGW_LINDr1] -> bus_selector53/1
  bus_selector53/1 -> SWCSetdownSta/1(SWC_Set_down_Sta)  "<CAN4_SWC_Set_down_Sta>"
  SWCSetdownSta/1(VHAL_SWCSetdownSta_flg) -> VHAL_SWCSetdownSta_flg/1
  [DT_CAN4_SG_zGW_LINDr1] -> bus_selector54/1
  bus_selector54/1 -> SWCTripSta/1(SWC_Trip_Sta)  "<CAN4_SWC_Trip_Sta>"
  SWCTripSta/1(VHAL_SWCTripSta_flg) -> VHAL_SWCTripSta_flg/1
  [DT_CAN4_SG_zGW_LINDr1] -> bus_selector55/1
  bus_selector55/1 -> SWCUndefinedSta/1(SWC_Undefined_Sta)  "<CAN4_SWC_Undefined_Sta>"
  SWCUndefinedSta/1(VHAL_SWCUndefinedSta_flg) -> VHAL_SWCUndefinedSta_flg/1
  [DT_CAN4_SG_zGW_LINDr1] -> bus_selector56/1
  bus_selector56/1 -> SWCUpSta/1(SWC_Up_Sta)  "<CAN4_SWC_Up_Sta>"
  SWCUpSta/1(VHAL_SWCUpSta_flg) -> VHAL_SWCUpSta_flg/1
  [DT_CAN4_SG_zGW_LINDr1] -> bus_selector57/1
  bus_selector57/1 -> SWCVRSta/1(SWC_VR_Sta)  "<CAN4_SWC_VR_Sta>"
  SWCVRSta/1(VHAL_SWCVRSta_flg) -> VHAL_SWCVRSta_flg/1
  [DT_CAN4_SG_zGW_LINDr1] -> bus_selector58/1
  bus_selector58/1 -> SWCmodeSta/1(SWC_mode_Sta)  "<CAN4_SWC_mode_Sta>"
  SWCmodeSta/1(VHAL_SWCmodeSta_flg) -> VHAL_SWCmodeSta_flg/1

== system halin/HAL_IN/CAN4/zGW_LINFr1 ==
  DT_CAN4_SG_zGW_LINFr1 : Inport
  AGSActualPosition : Subsystem
  bus_selector : BusSelector  OutputSignals=CAN4_AGS_Actual_Position
  VHAL_AGSActualPosition_enum : Outport
  wires:
  DT_CAN4_SG_zGW_LINFr1/1 -> [DT_CAN4_SG_zGW_LINFr1]
  [DT_CAN4_SG_zGW_LINFr1] -> bus_selector/1
  bus_selector/1 -> AGSActualPosition/1(AGS_Actual_Position)  "<CAN4_AGS_Actual_Position>"
  AGSActualPosition/1(VHAL_AGSActualPosition_enum) -> VHAL_AGSActualPosition_enum/1

== system halin/HAL_IN/CAN4/zGW_SEAT1 ==
  DT_CAN4_SG_zGW_SEAT1 : Inport
  DSEATAntiSta : Subsystem
  DSEATEntryFunSta : Subsystem
  DSEATErrorSta : Subsystem
  DSEATHWVer : Subsystem
  DSEATMode : Subsystem
  DSEATSWVer : Subsystem
  DSEATVentSta : Subsystem
  DSEATheatersta : Subsystem
  PSEATErrorSta : Subsystem
  PSEATHWVer : Subsystem
  PSEATMode : Subsystem
  PSEATSWVer : Subsystem
  PSEATVentSta : Subsystem
  PSEATheatersta : Subsystem
  bus_selector : BusSelector  OutputSignals=CAN4_DSEAT_Anti_Sta
  bus_selector1 : BusSelector  OutputSignals=CAN4_DSEAT_EntryFun_Sta
  bus_selector10 : BusSelector  OutputSignals=CAN4_PSEAT_Mode
  bus_selector11 : BusSelector  OutputSignals=CAN4_PSEAT_SW_Ver
  bus_selector12 : BusSelector  OutputSignals=CAN4_PSEAT_Vent_Sta
  bus_selector13 : BusSelector  OutputSignals=CAN4_PSEAT_heater_sta
  bus_selector2 : BusSelector  OutputSignals=CAN4_DSEAT_Error_Sta
  bus_selector3 : BusSelector  OutputSignals=CAN4_DSEAT_HW_Ver
  bus_selector4 : BusSelector  OutputSignals=CAN4_DSEAT_Mode
  bus_selector5 : BusSelector  OutputSignals=CAN4_DSEAT_SW_Ver
  bus_selector6 : BusSelector  OutputSignals=CAN4_DSEAT_Vent_Sta
  bus_selector7 : BusSelector  OutputSignals=CAN4_DSEAT_heater_sta
  bus_selector8 : BusSelector  OutputSignals=CAN4_PSEAT_Error_Sta
  bus_selector9 : BusSelector  OutputSignals=CAN4_PSEAT_HW_Ver
  VHAL_DSEATAntiSta_flg : Outport
  VHAL_DSEATEntryFunSta_flg : Outport  Port=2
  VHAL_DSEATErrorSta_flg : Outport  Port=3
  VHAL_DSEATHWVer_enum : Outport  Port=4
  VHAL_DSEATMode_enum : Outport  Port=5
  VHAL_DSEATSWVer_enum : Outport  Port=6
  VHAL_DSEATVentSta_enum : Outport  Port=7
  VHAL_DSEATheatersta_enum : Outport  Port=8
  VHAL_PSEATErrorSta_flg : Outport  Port=9
  VHAL_PSEATHWVer_enum : Outport  Port=10
  VHAL_PSEATMode_enum : Outport  Port=11
  VHAL_PSEATSWVer_enum : Outport  Port=12
  VHAL_PSEATVentSta_enum : Outport  Port=13
  VHAL_PSEATheatersta_enum : Outport  Port=14
  wires:
  DT_CAN4_SG_zGW_SEAT1/1 -> [DT_CAN4_SG_zGW_SEAT1]
  [DT_CAN4_SG_zGW_SEAT1] -> bus_selector/1
  bus_selector/1 -> DSEATAntiSta/1(DSEAT_Anti_Sta)  "<CAN4_DSEAT_Anti_Sta>"
  DSEATAntiSta/1(VHAL_DSEATAntiSta_flg) -> VHAL_DSEATAntiSta_flg/1
  [DT_CAN4_SG_zGW_SEAT1] -> bus_selector1/1
  bus_selector1/1 -> DSEATEntryFunSta/1(DSEAT_EntryFun_Sta)  "<CAN4_DSEAT_EntryFun_Sta>"
  DSEATEntryFunSta/1(VHAL_DSEATEntryFunSta_flg) -> VHAL_DSEATEntryFunSta_flg/1
  [DT_CAN4_SG_zGW_SEAT1] -> bus_selector2/1
  bus_selector2/1 -> DSEATErrorSta/1(DSEAT_Error_Sta)  "<CAN4_DSEAT_Error_Sta>"
  DSEATErrorSta/1(VHAL_DSEATErrorSta_flg) -> VHAL_DSEATErrorSta_flg/1
  [DT_CAN4_SG_zGW_SEAT1] -> bus_selector3/1
  bus_selector3/1 -> DSEATHWVer/1(DSEAT_HW_Ver)  "<CAN4_DSEAT_HW_Ver>"
  DSEATHWVer/1(VHAL_DSEATHWVer_enum) -> VHAL_DSEATHWVer_enum/1
  [DT_CAN4_SG_zGW_SEAT1] -> bus_selector4/1
  bus_selector4/1 -> DSEATMode/1(DSEAT_Mode)  "<CAN4_DSEAT_Mode>"
  DSEATMode/1(VHAL_DSEATMode_enum) -> VHAL_DSEATMode_enum/1
  [DT_CAN4_SG_zGW_SEAT1] -> bus_selector5/1
  bus_selector5/1 -> DSEATSWVer/1(DSEAT_SW_Ver)  "<CAN4_DSEAT_SW_Ver>"
  DSEATSWVer/1(VHAL_DSEATSWVer_enum) -> VHAL_DSEATSWVer_enum/1
  [DT_CAN4_SG_zGW_SEAT1] -> bus_selector6/1
  bus_selector6/1 -> DSEATVentSta/1(DSEAT_Vent_Sta)  "<CAN4_DSEAT_Vent_Sta>"
  DSEATVentSta/1(VHAL_DSEATVentSta_enum) -> VHAL_DSEATVentSta_enum/1
  [DT_CAN4_SG_zGW_SEAT1] -> bus_selector7/1
  bus_selector7/1 -> DSEATheatersta/1(DSEAT_heater_sta)  "<CAN4_DSEAT_heater_sta>"
  DSEATheatersta/1(VHAL_DSEATheatersta_enum) -> VHAL_DSEATheatersta_enum/1
  [DT_CAN4_SG_zGW_SEAT1] -> bus_selector8/1
  bus_selector8/1 -> PSEATErrorSta/1(PSEAT_Error_Sta)  "<CAN4_PSEAT_Error_Sta>"
  PSEATErrorSta/1(VHAL_PSEATErrorSta_flg) -> VHAL_PSEATErrorSta_flg/1
  [DT_CAN4_SG_zGW_SEAT1] -> bus_selector9/1
  bus_selector9/1 -> PSEATHWVer/1(PSEAT_HW_Ver)  "<CAN4_PSEAT_HW_Ver>"
  PSEATHWVer/1(VHAL_PSEATHWVer_enum) -> VHAL_PSEATHWVer_enum/1
  [DT_CAN4_SG_zGW_SEAT1] -> bus_selector10/1
  bus_selector10/1 -> PSEATMode/1(PSEAT_Mode)  "<CAN4_PSEAT_Mode>"
  PSEATMode/1(VHAL_PSEATMode_enum) -> VHAL_PSEATMode_enum/1
  [DT_CAN4_SG_zGW_SEAT1] -> bus_selector11/1
  bus_selector11/1 -> PSEATSWVer/1(PSEAT_SW_Ver)  "<CAN4_PSEAT_SW_Ver>"
  PSEATSWVer/1(VHAL_PSEATSWVer_enum) -> VHAL_PSEATSWVer_enum/1
  [DT_CAN4_SG_zGW_SEAT1] -> bus_selector12/1
  bus_selector12/1 -> PSEATVentSta/1(PSEAT_Vent_Sta)  "<CAN4_PSEAT_Vent_Sta>"
  PSEATVentSta/1(VHAL_PSEATVentSta_enum) -> VHAL_PSEATVentSta_enum/1
  [DT_CAN4_SG_zGW_SEAT1] -> bus_selector13/1
  bus_selector13/1 -> PSEATheatersta/1(PSEAT_heater_sta)  "<CAN4_PSEAT_heater_sta>"
  PSEATheatersta/1(VHAL_PSEATheatersta_enum) -> VHAL_PSEATheatersta_enum/1

== system halin/HAL_IN/CAN5/TBOX1 ==
  DT_CAN5_SG_TBOX1 : Inport
  CbnPreACEnaReq : Subsystem
  PowerOffTSet : Subsystem
  ReDoorLock : Subsystem
  ReOutsideMirror : Subsystem
  RePwrReqTbox : Subsystem
  ReRadio : Subsystem
  RemoteACTemp : Subsystem
  RemoteAutoReq : Subsystem
  TBOXNETSIGSTR : Subsystem
  TBOXRemotePW : Subsystem
  TBOXTESTSTATUS : Subsystem
  bus_selector : BusSelector  OutputSignals=CAN5_CbnPreACEnaReq
  bus_selector1 : BusSelector  OutputSignals=CAN5_PowerOff_T_Set
  bus_selector10 : BusSelector  OutputSignals=CAN5_TBOX_TEST_STATUS
  bus_selector2 : BusSelector  OutputSignals=CAN5_ReOutsideMirror
  bus_selector3 : BusSelector  OutputSignals=CAN5_Re_DoorLock
  bus_selector4 : BusSelector  OutputSignals=CAN5_Re_PwrReqTbox
  bus_selector5 : BusSelector  OutputSignals=CAN5_Re_Radio
  bus_selector6 : BusSelector  OutputSignals=CAN5_Remote_ACTemp
  bus_selector7 : BusSelector  OutputSignals=CAN5_Remote_AutoReq
  bus_selector8 : BusSelector  OutputSignals=CAN5_TBOX_NET_SIG_STR
  bus_selector9 : BusSelector  OutputSignals=CAN5_TBOX_Remote_PW
  VHAL_CbnPreACEnaReq_enum : Outport
  VHAL_PowerOffTSet_cnt : Outport  Port=2
  VHAL_ReOutsideMirror_enum : Outport  Port=3
  VHAL_ReDoorLock_enum : Outport  Port=4
  VHAL_RePwrReqTbox_enum : Outport  Port=5
  VHAL_ReRadio_flg : Outport  Port=6
  VHAL_RemoteACTemp_C : Outport  Port=7
  VHAL_RemoteAutoReq_flg : Outport  Port=8
  VHAL_TBOXNETSIGSTR_enum : Outport  Port=9
  VHAL_TBOXRemotePW_enum : Outport  Port=10
  VHAL_TBOXTESTSTATUS_enum : Outport  Port=11
  wires:
  DT_CAN5_SG_TBOX1/1 -> [DT_CAN5_SG_TBOX1]
  [DT_CAN5_SG_TBOX1] -> bus_selector/1
  bus_selector/1 -> CbnPreACEnaReq/1(CbnPreACEnaReq)  "<CAN5_CbnPreACEnaReq>"
  CbnPreACEnaReq/1(VHAL_CbnPreACEnaReq_enum) -> VHAL_CbnPreACEnaReq_enum/1
  [DT_CAN5_SG_TBOX1] -> bus_selector1/1
  bus_selector1/1 -> PowerOffTSet/1(PowerOff_T_Set)  "<CAN5_PowerOff_T_Set>"
  PowerOffTSet/1(VHAL_PowerOffTSet_cnt) -> VHAL_PowerOffTSet_cnt/1
  [DT_CAN5_SG_TBOX1] -> bus_selector2/1
  bus_selector2/1 -> ReOutsideMirror/1(ReOutsideMirror)  "<CAN5_ReOutsideMirror>"
  ReOutsideMirror/1(VHAL_ReOutsideMirror_enum) -> VHAL_ReOutsideMirror_enum/1
  [DT_CAN5_SG_TBOX1] -> bus_selector3/1
  bus_selector3/1 -> ReDoorLock/1(Re_DoorLock)  "<CAN5_Re_DoorLock>"
  ReDoorLock/1(VHAL_ReDoorLock_enum) -> VHAL_ReDoorLock_enum/1
  [DT_CAN5_SG_TBOX1] -> bus_selector4/1
  bus_selector4/1 -> RePwrReqTbox/1(Re_PwrReqTbox)  "<CAN5_Re_PwrReqTbox>"
  RePwrReqTbox/1(VHAL_RePwrReqTbox_enum) -> VHAL_RePwrReqTbox_enum/1
  [DT_CAN5_SG_TBOX1] -> bus_selector5/1
  bus_selector5/1 -> ReRadio/1(Re_Radio)  "<CAN5_Re_Radio>"
  ReRadio/1(VHAL_ReRadio_flg) -> VHAL_ReRadio_flg/1
  [DT_CAN5_SG_TBOX1] -> bus_selector6/1
  bus_selector6/1 -> RemoteACTemp/1(Remote_ACTemp)  "<CAN5_Remote_ACTemp>"
  RemoteACTemp/1(VHAL_RemoteACTemp_C) -> VHAL_RemoteACTemp_C/1
  [DT_CAN5_SG_TBOX1] -> bus_selector7/1
  bus_selector7/1 -> RemoteAutoReq/1(Remote_AutoReq)  "<CAN5_Remote_AutoReq>"
  RemoteAutoReq/1(VHAL_RemoteAutoReq_flg) -> VHAL_RemoteAutoReq_flg/1
  [DT_CAN5_SG_TBOX1] -> bus_selector8/1
  bus_selector8/1 -> TBOXNETSIGSTR/1(TBOX_NET_SIG_STR)  "<CAN5_TBOX_NET_SIG_STR>"
  TBOXNETSIGSTR/1(VHAL_TBOXNETSIGSTR_enum) -> VHAL_TBOXNETSIGSTR_enum/1
  [DT_CAN5_SG_TBOX1] -> bus_selector9/1
  bus_selector9/1 -> TBOXRemotePW/1(TBOX_Remote_PW)  "<CAN5_TBOX_Remote_PW>"
  TBOXRemotePW/1(VHAL_TBOXRemotePW_enum) -> VHAL_TBOXRemotePW_enum/1
  [DT_CAN5_SG_TBOX1] -> bus_selector10/1
  bus_selector10/1 -> TBOXTESTSTATUS/1(TBOX_TEST_STATUS)  "<CAN5_TBOX_TEST_STATUS>"
  TBOXTESTSTATUS/1(VHAL_TBOXTESTSTATUS_enum) -> VHAL_TBOXTESTSTATUS_enum/1

== system halin/HAL_IN/CAN5/TBOX2 ==
  DT_CAN5_SG_TBOX2 : Inport
  TimeSyncFromBSDay : Subsystem
  TimeSyncFromBSHour : Subsystem
  TimeSyncFromBSMinute : Subsystem
  TimeSyncFromBSMonth : Subsystem
  TimeSyncFromBSSecond : Subsystem
  TimeSyncFromBSYear : Subsystem
  bus_selector : BusSelector  OutputSignals=CAN5_TimeSyncFromBS_Day
  bus_selector1 : BusSelector  OutputSignals=CAN5_TimeSyncFromBS_Hour
  bus_selector2 : BusSelector  OutputSignals=CAN5_TimeSyncFromBS_Minute
  bus_selector3 : BusSelector  OutputSignals=CAN5_TimeSyncFromBS_Month
  bus_selector4 : BusSelector  OutputSignals=CAN5_TimeSyncFromBS_Second
  bus_selector5 : BusSelector  OutputSignals=CAN5_TimeSyncFromBS_Year
  VHAL_TimeSyncFromBSDay_DAY : Outport
  VHAL_TimeSyncFromBSHour_hr : Outport  Port=2
  VHAL_TimeSyncFromBSMinute_min : Outport  Port=3
  VHAL_TimeSyncFromBSMonth_MONTH : Outport  Port=4
  VHAL_TimeSyncFromBSSecond_s : Outport  Port=5
  VHAL_TimeSyncFromBSYear_YEAR : Outport  Port=6
  wires:
  DT_CAN5_SG_TBOX2/1 -> [DT_CAN5_SG_TBOX2]
  [DT_CAN5_SG_TBOX2] -> bus_selector/1
  bus_selector/1 -> TimeSyncFromBSDay/1(TimeSyncFromBS_Day)  "<CAN5_TimeSyncFromBS_Day>"
  TimeSyncFromBSDay/1(VHAL_TimeSyncFromBSDay_DAY) -> VHAL_TimeSyncFromBSDay_DAY/1
  [DT_CAN5_SG_TBOX2] -> bus_selector1/1
  bus_selector1/1 -> TimeSyncFromBSHour/1(TimeSyncFromBS_Hour)  "<CAN5_TimeSyncFromBS_Hour>"
  TimeSyncFromBSHour/1(VHAL_TimeSyncFromBSHour_hr) -> VHAL_TimeSyncFromBSHour_hr/1
  [DT_CAN5_SG_TBOX2] -> bus_selector2/1
  bus_selector2/1 -> TimeSyncFromBSMinute/1(TimeSyncFromBS_Minute)  "<CAN5_TimeSyncFromBS_Minute>"
  TimeSyncFromBSMinute/1(VHAL_TimeSyncFromBSMinute_min) -> VHAL_TimeSyncFromBSMinute_min/1
  [DT_CAN5_SG_TBOX2] -> bus_selector3/1
  bus_selector3/1 -> TimeSyncFromBSMonth/1(TimeSyncFromBS_Month)  "<CAN5_TimeSyncFromBS_Month>"
  TimeSyncFromBSMonth/1(VHAL_TimeSyncFromBSMonth_MONTH) -> VHAL_TimeSyncFromBSMonth_MONTH/1
  [DT_CAN5_SG_TBOX2] -> bus_selector4/1
  bus_selector4/1 -> TimeSyncFromBSSecond/1(TimeSyncFromBS_Second)  "<CAN5_TimeSyncFromBS_Second>"
  TimeSyncFromBSSecond/1(VHAL_TimeSyncFromBSSecond_s) -> VHAL_TimeSyncFromBSSecond_s/1
  [DT_CAN5_SG_TBOX2] -> bus_selector5/1
  bus_selector5/1 -> TimeSyncFromBSYear/1(TimeSyncFromBS_Year)  "<CAN5_TimeSyncFromBS_Year>"
  TimeSyncFromBSYear/1(VHAL_TimeSyncFromBSYear_YEAR) -> VHAL_TimeSyncFromBSYear_YEAR/1

== system halin/HAL_IN/CAN5/TBOX3 ==
  DT_CAN5_SG_TBOX3 : Inport
  ChargePercentSet : Subsystem
  ReserveChargeOFFDay : Subsystem
  ReserveChargeOFFHour : Subsystem
  ReserveChargeOFFMinute : Subsystem
  ReserveChargeOFFMonth : Subsystem
  ReserveChargeOFFYear : Subsystem
  ReserveChargeOnDay : Subsystem
  ReserveChargeOnHour : Subsystem
  ReserveChargeOnMinute : Subsystem
  ReserveChargeOnMonth : Subsystem
  ReserveChargeOnYear : Subsystem
  TBOXHWVER : Subsystem
  TBOXSWVER : Subsystem
  bus_selector : BusSelector  OutputSignals=CAN5_Charge_Percent_Set
  bus_selector1 : BusSelector  OutputSignals=CAN5_ReserveChargeOFF_Day
  bus_selector10 : BusSelector  OutputSignals=CAN5_ReserveChargeOn_Year
  bus_selector11 : BusSelector  OutputSignals=CAN5_TBOX_HW_VER
  bus_selector12 : BusSelector  OutputSignals=CAN5_TBOX_SW_VER
  bus_selector2 : BusSelector  OutputSignals=CAN5_ReserveChargeOFF_Hour
  bus_selector3 : BusSelector  OutputSignals=CAN5_ReserveChargeOFF_Minute
  bus_selector4 : BusSelector  OutputSignals=CAN5_ReserveChargeOFF_Month
  bus_selector5 : BusSelector  OutputSignals=CAN5_ReserveChargeOFF_Year
  bus_selector6 : BusSelector  OutputSignals=CAN5_ReserveChargeOn_Day
  bus_selector7 : BusSelector  OutputSignals=CAN5_ReserveChargeOn_Hour
  bus_selector8 : BusSelector  OutputSignals=CAN5_ReserveChargeOn_Minute
  bus_selector9 : BusSelector  OutputSignals=CAN5_ReserveChargeOn_Month
  VHAL_ChargePercentSet_pct : Outport
  VHAL_ReserveChargeOFFDay_DAY : Outport  Port=2
  VHAL_ReserveChargeOFFHour_hr : Outport  Port=3
  VHAL_ReserveChargeOFFMinute_min : Outport  Port=4
  VHAL_ReserveChargeOFFMonth_MONTH : Outport  Port=5
  VHAL_ReserveChargeOFFYear_YEAR : Outport  Port=6
  VHAL_ReserveChargeOnDay_DAY : Outport  Port=7
  VHAL_ReserveChargeOnHour_hr : Outport  Port=8
  VHAL_ReserveChargeOnMinute_min : Outport  Port=9
  VHAL_ReserveChargeOnMonth_MONTH : Outport  Port=10
  VHAL_ReserveChargeOnYear_YEAR : Outport  Port=11
  VHAL_TBOXHWVER_enum : Outport  Port=12
  VHAL_TBOXSWVER_enum : Outport  Port=13
  wires:
  DT_CAN5_SG_TBOX3/1 -> [DT_CAN5_SG_TBOX3]
  [DT_CAN5_SG_TBOX3] -> bus_selector/1
  bus_selector/1 -> ChargePercentSet/1(Charge_Percent_Set)  "<CAN5_Charge_Percent_Set>"
  ChargePercentSet/1(VHAL_ChargePercentSet_pct) -> VHAL_ChargePercentSet_pct/1
  [DT_CAN5_SG_TBOX3] -> bus_selector1/1
  bus_selector1/1 -> ReserveChargeOFFDay/1(ReserveChargeOFF_Day)  "<CAN5_ReserveChargeOFF_Day>"
  ReserveChargeOFFDay/1(VHAL_ReserveChargeOFFDay_DAY) -> VHAL_ReserveChargeOFFDay_DAY/1
  [DT_CAN5_SG_TBOX3] -> bus_selector2/1
  bus_selector2/1 -> ReserveChargeOFFHour/1(ReserveChargeOFF_Hour)  "<CAN5_ReserveChargeOFF_Hour>"
  ReserveChargeOFFHour/1(VHAL_ReserveChargeOFFHour_hr) -> VHAL_ReserveChargeOFFHour_hr/1
  [DT_CAN5_SG_TBOX3] -> bus_selector3/1
  bus_selector3/1 -> ReserveChargeOFFMinute/1(ReserveChargeOFF_Minute)  "<CAN5_ReserveChargeOFF_Minute>"
  ReserveChargeOFFMinute/1(VHAL_ReserveChargeOFFMinute_min) -> VHAL_ReserveChargeOFFMinute_min/1
  [DT_CAN5_SG_TBOX3] -> bus_selector4/1
  bus_selector4/1 -> ReserveChargeOFFMonth/1(ReserveChargeOFF_Month)  "<CAN5_ReserveChargeOFF_Month>"
  ReserveChargeOFFMonth/1(VHAL_ReserveChargeOFFMonth_MONTH) -> VHAL_ReserveChargeOFFMonth_MONTH/1
  [DT_CAN5_SG_TBOX3] -> bus_selector5/1
  bus_selector5/1 -> ReserveChargeOFFYear/1(ReserveChargeOFF_Year)  "<CAN5_ReserveChargeOFF_Year>"
  ReserveChargeOFFYear/1(VHAL_ReserveChargeOFFYear_YEAR) -> VHAL_ReserveChargeOFFYear_YEAR/1
  [DT_CAN5_SG_TBOX3] -> bus_selector6/1
  bus_selector6/1 -> ReserveChargeOnDay/1(ReserveChargeOn_Day)  "<CAN5_ReserveChargeOn_Day>"
  ReserveChargeOnDay/1(VHAL_ReserveChargeOnDay_DAY) -> VHAL_ReserveChargeOnDay_DAY/1
  [DT_CAN5_SG_TBOX3] -> bus_selector7/1
  bus_selector7/1 -> ReserveChargeOnHour/1(ReserveChargeOn_Hour)  "<CAN5_ReserveChargeOn_Hour>"
  ReserveChargeOnHour/1(VHAL_ReserveChargeOnHour_hr) -> VHAL_ReserveChargeOnHour_hr/1
  [DT_CAN5_SG_TBOX3] -> bus_selector8/1
  bus_selector8/1 -> ReserveChargeOnMinute/1(ReserveChargeOn_Minute)  "<CAN5_ReserveChargeOn_Minute>"
  ReserveChargeOnMinute/1(VHAL_ReserveChargeOnMinute_min) -> VHAL_ReserveChargeOnMinute_min/1
  [DT_CAN5_SG_TBOX3] -> bus_selector9/1
  bus_selector9/1 -> ReserveChargeOnMonth/1(ReserveChargeOn_Month)  "<CAN5_ReserveChargeOn_Month>"
  ReserveChargeOnMonth/1(VHAL_ReserveChargeOnMonth_MONTH) -> VHAL_ReserveChargeOnMonth_MONTH/1
  [DT_CAN5_SG_TBOX3] -> bus_selector10/1
  bus_selector10/1 -> ReserveChargeOnYear/1(ReserveChargeOn_Year)  "<CAN5_ReserveChargeOn_Year>"
  ReserveChargeOnYear/1(VHAL_ReserveChargeOnYear_YEAR) -> VHAL_ReserveChargeOnYear_YEAR/1
  [DT_CAN5_SG_TBOX3] -> bus_selector11/1
  bus_selector11/1 -> TBOXHWVER/1(TBOX_HW_VER)  "<CAN5_TBOX_HW_VER>"
  TBOXHWVER/1(VHAL_TBOXHWVER_enum) -> VHAL_TBOXHWVER_enum/1
  [DT_CAN5_SG_TBOX3] -> bus_selector12/1
  bus_selector12/1 -> TBOXSWVER/1(TBOX_SW_VER)  "<CAN5_TBOX_SW_VER>"
  TBOXSWVER/1(VHAL_TBOXSWVER_enum) -> VHAL_TBOXSWVER_enum/1
